simulink model "Two_Attitude_Estimation_ekf"  (R2021a)
settings: Solver=FixedStepAuto  StartTime=0.0  StopTime=200  FixedStep=Ts  RelTol=1e-5
values from neighbouring files (symbols this model uses):
  accel_filter_coef = [    0.0264    0.1405    0.3331    0.3331    0.1405    0.0264]    [quad_params_ekf.m]
  g = ref_acc(3)    [ekf_measurement_jacobian.m]    (also in quad_params_ekf.m = 9.81)
  gyro_filter_den = [ 1.0000    2.2287    2.5245    1.5773    0.5410    0.0796]    [quad_params_ekf.m]
  gyro_filter_num = [ 0.2821    1.2725    2.4208    2.4208    1.2725    0.2821]    [quad_params_ekf.m]
  I = [     0.005831943165131                   0                   0 ... (first row only)    [quad_params_ekf.m]
  Kd_rates = [0.05,0.05,0.1]'    [quad_params_ekf.m]
  Kd_vel = [0.8,0.8,0.3]'    [quad_params_ekf.m]
  Ki_vel = [0.1,0.1,0.1]'    [quad_params_ekf.m]
  km = 1.2e-7    (= 1.2e-07)    [quad_params_ekf.m]
  Kp_att = [6,6,6]'    [quad_params_ekf.m]
  Kp_pos = [7,7,3]'    [quad_params_ekf.m]
  Kp_rates = [10,10,10]'    [quad_params_ekf.m]
  Kp_vel = [3,3,5]'    [quad_params_ekf.m]
  kt = 0.9e-5    (= 9e-06)    [quad_params_ekf.m]
  L = 0.2    [quad_params_ekf.m]
  m = 0.9272    [quad_params_ekf.m]
  P_init = 0.01*eye(7)    [quad_params_ekf.m]
  Q = diag([0.015,0.0150,0.0150,0.0150,0.001,0.001,0.001])    [quad_params_ekf.m]
  q_init = [1;0;0;0]    [quad_params_ekf.m]
  R = diag([0.35,0.35,0.35,0.05,0.05,0.05])    [quad_params_ekf.m]
  rate_p_max = 3.5    [quad_params_ekf.m]
  thrust_max = thrust_max_per_motor*4    (= 32)    [quad_params_ekf.m]
  thrust_max_per_motor = 8    [quad_params_ekf.m]
  tilt_max = pi/6    (= 0.523598775598)    [quad_params_ekf.m]
  TQ_max_per_motor = km*(w_max.^2)    [quad_params_ekf.m]
  Ts = 0.001    [ekf_process_jacobian.m]    (also in ekf_process_model.m; quad_params_ekf.m)
  Ts_IMU = 0.001    [quad_params_ekf.m]
  Vb_init = [0;0;0]    [quad_params_ekf.m]
  vel_xy_max = 15    [quad_params_ekf.m]
  vel_z_max = 10    [quad_params_ekf.m]
  wb_init = [0;0;0]    [quad_params_ekf.m]
  x_0 = [1 0 0 0 0 0 0]'    [quad_params_ekf.m]
  Xe_init = [0;0;0]    [quad_params_ekf.m]
undefined symbols (not defined in the file or in its folder): IMU, p, pm_0, sigbuilder_block, Vm_0, xme_0
libraries: aerolibutil x8, simulink_extras x8, sharedtransform x7, sharedutil x6, simulink x4, pid_lib x3, aerolibcommonsys x3, aerolibnavsys x2, dspstat3 x2, mspsensorlib x1, aerolibnav x1, dspmtrx3 x1
(part 2 of 4)

== system Two_Attitude_Estimation_ekf/Thrust to attitude ==
  note: Thrust vector and Yaw to Attitude and total Thrust
  thrust_sp : Inport
  yaw_sp : Inport  Port=2
  Bus Creator : BusCreator  Inputs=3
  Demux4 : Demux  Outputs=3
  Direction Cosine Matrix to Quaternions : sharedtransform/Direction Cosine Matrix  to Quaternions  aMode=0  action=None  tolerance=eps(2)
      settings: SourceProductBaseCode=AE,PW,DR,MT,UV,VE
  MATLAB Function4 : MATLAB Function  TreatAsAtomicUnit=on
  Quaternions to Rotation Angles : sharedtransform/Quaternions to Rotation Angles  rotationOrder=ZYX  aMode=aMode
      settings: SourceProductBaseCode=AE,PW,DR,MT,UV,VE
  Scope1 : Scope
  Scope2 : Scope
  To Workspace : ToWorkspace  VariableName=thrust_unit_dir  SaveFormat=Timeseries  SampleTime=-1
  To Workspace1 : ToWorkspace  VariableName=thrust_mag  SaveFormat=Timeseries  SampleTime=-1
  thrust_mag : Outport
  q_cmd : Outport  Port=2
  euler_cmd : Outport  Port=3
  wires:
  thrust_sp/1 -> Scope1/1, MATLAB Function4/1(thrust_sp)  "thrust_cmd"
  MATLAB Function4/1(R_sp) -> To Workspace/1, Direction Cosine Matrix to Quaternions/1
  MATLAB Function4/2(thrust_mag) -> thrust_mag/1, To Workspace1/1
  Direction Cosine Matrix to Quaternions/1 -> q_cmd/1, Quaternions to Rotation Angles/1
  yaw_sp/1 -> MATLAB Function4/2(yaw_sp)  "yaw_cmd"
  Demux4/1 -> Bus Creator/1  "yaw"
  Demux4/3 -> Bus Creator/3  "roll"
  Bus Creator/1 -> Scope2/1, euler_cmd/1
  Demux4/2 -> Bus Creator/2  "pitch"
  Quaternions to Rotation Angles/1 -> Demux4/1

== system Two_Attitude_Estimation_ekf/Trajectory command ==
  Altitude : Subsystem  VariantControl=1
  Ground : Subsystem  VariantControl=0
  Position Trajectory : Subsystem  VariantControl=5
  Test to visualize thrust dir : Subsystem  VariantControl=6
  X Sine : Subsystem  VariantControl=4
  X ramp : Subsystem  VariantControl=9
  X square : Subsystem  VariantControl=7
  Y Sine : Subsystem  VariantControl=3
  Y ramp : Subsystem  VariantControl=8
  Yaw Sine : Subsystem  VariantControl=2
  Yaw steps : Subsystem  VariantControl=10
  Z : Outport
  Y : Outport  Port=2
  X : Outport  Port=3
  Yaw : Outport  Port=4
  CMD_VEC : Outport  Port=5

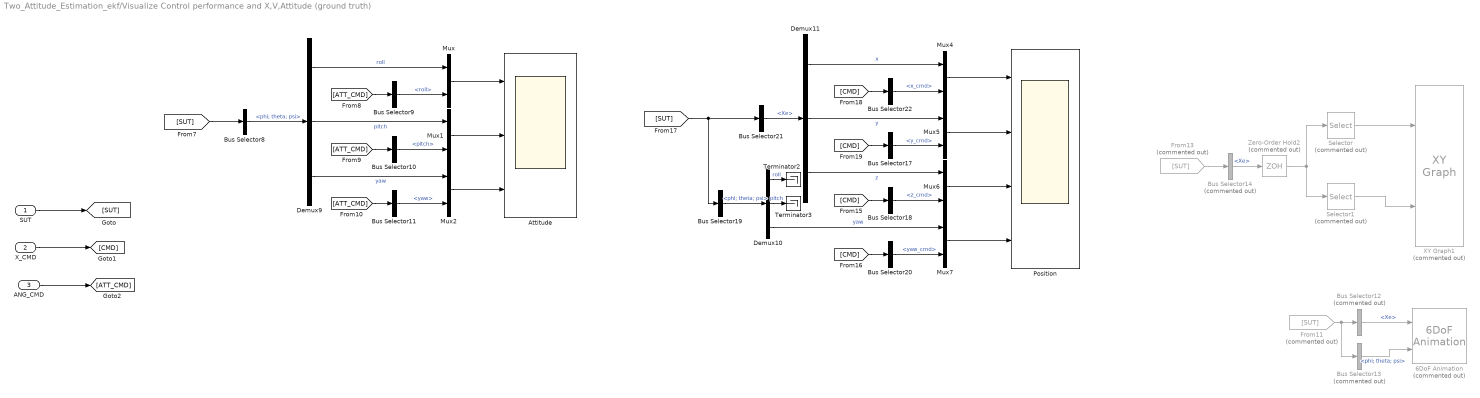
== system Two_Attitude_Estimation_ekf/Visualize Control performance and X,V,Attitude (ground truth) ==
  SUT : Inport
  X_CMD : Inport  Port=2
  ANG_CMD : Inport  Port=3
  6DoF Animation : aerolibanim/6DoF Animation  Commented=on  u1=[-20 20 -20 20 -20 20]  u2=0.05  u3=0.5  u4=[-5 -5 0 5]  u5=Fly alongside  u6=[0 0 0]  u7=10  u8=on
  "Attitude " : Scope  NumInputPorts=3
  Bus Selector10 : BusSelector  OutputSignals=pitch
  Bus Selector11 : BusSelector  OutputSignals=yaw
  Bus Selector12 : BusSelector  Commented=on  OutputSignals=Xe
  Bus Selector13 : BusSelector  Commented=on  OutputSignals=phi; theta; psi
  Bus Selector14 : BusSelector  Commented=on  OutputSignals=Xe
  Bus Selector17 : BusSelector  OutputSignals=y_cmd
  Bus Selector18 : BusSelector  OutputSignals=z_cmd
  Bus Selector19 : BusSelector  OutputSignals=phi; theta; psi
  Bus Selector20 : BusSelector  OutputSignals=yaw_cmd
  Bus Selector21 : BusSelector  OutputSignals=Xe
  Bus Selector22 : BusSelector  OutputSignals=x_cmd
  Bus Selector8 : BusSelector  OutputSignals=phi; theta; psi
  Bus Selector9 : BusSelector  OutputSignals=roll
  Demux10 : Demux  Outputs=3
  Demux11 : Demux  Outputs=3
  Demux9 : Demux  Outputs=3
  From11 : From  Commented=on  GotoTag=SUT
  From13 : From  Commented=on  GotoTag=SUT
  Mux{,1..2,4..7} (7 alike) : Mux  Inputs=2
  Position : Scope  NumInputPorts=4
  Selector : Selector  Commented=on  InputPortWidth=3  IndexOptions=Index vector (dialog)  Indices=1  OutputSizes=1
  Selector1 : Selector  Commented=on  InputPortWidth=3  IndexOptions=Index vector (dialog)  Indices=2  OutputSizes=1
  Terminator2 : Terminator
  Terminator3 : Terminator
  XY Graph1 : simulink/Sinks/XY Graph  Commented=on  xmin=-1  xmax=30  ymin=-1  ymax=35  st=-1
  Zero-Order Hold2 : ZeroOrderHold  Commented=on  SampleTime=0.1
  wires:
  SUT/1 -> [SUT]
  X_CMD/1 -> [CMD]
  [SUT] -> Bus Selector8/1
  Demux9/2 -> Mux1/1  "pitch"
  Demux9/1 -> Mux/1  "roll"
  Bus Selector8/1 -> Demux9/1  "<phi; theta; psi>"
  Mux/1 -> "Attitude "/1
  Mux1/1 -> "Attitude "/2
  Mux2/1 -> "Attitude "/3
  Demux9/3 -> Mux2/1  "yaw"
  [ATT_CMD] -> Bus Selector9/1
  Bus Selector9/1 -> Mux/2  "<roll>"
  [ATT_CMD] -> Bus Selector10/1
  Bus Selector10/1 -> Mux1/2  "<pitch>"
  [ATT_CMD] -> Bus Selector11/1
  Bus Selector11/1 -> Mux2/2  "<yaw>"
  From13/1 -> Bus Selector14/1
  Bus Selector14/1 -> Zero-Order Hold2/1  "<Xe>"
  Zero-Order Hold2/1 -> Selector1/1, Selector/1
  Demux10/3 -> Mux7/1  "yaw"
  Mux7/1 -> Position/4
  Demux11/1 -> Mux4/1  "x"
  [CMD] -> Bus Selector20/1
  Bus Selector20/1 -> Mux7/2  "<yaw_cmd>"
  [CMD] -> Bus Selector17/1
  [SUT] -> Bus Selector21/1, Bus Selector19/1
  Demux10/2 -> Terminator3/1  "pitch"
  Mux6/1 -> Position/3
  Bus Selector19/1 -> Demux10/1  "<phi; theta; psi>"
  Demux10/1 -> Terminator2/1  "roll"
  Demux11/2 -> Mux5/1  "y"
  Bus Selector17/1 -> Mux5/2  "<y_cmd>"
  Mux4/1 -> Position/1
  Demux11/3 -> Mux6/1  "z"
  [CMD] -> Bus Selector22/1
  Mux5/1 -> Position/2
  Bus Selector22/1 -> Mux4/2  "<x_cmd>"
  Bus Selector18/1 -> Mux6/2  "<z_cmd>"
  [CMD] -> Bus Selector18/1
  Bus Selector21/1 -> Demux11/1  "<Xe>"
  ANG_CMD/1 -> [ATT_CMD]
  Selector/1 -> XY Graph1/1
  Selector1/1 -> XY Graph1/2
  From11/1 -> Bus Selector13/1, Bus Selector12/1
  Bus Selector12/1 -> 6DoF Animation/1  "<Xe>"
  Bus Selector13/1 -> 6DoF Animation/2  "<phi; theta; psi>"

== system Two_Attitude_Estimation_ekf/Control allocation and motor control/Ideal Actuators with allocation ==
  THRUST_CMD : Inport
  TQ_Roll_CMD : Inport  Port=2
  TQ_Pitch_CMD : Inport  Port=3
  TQ_Yaw_CMD : Inport  Port=4
  Control allocation : Subsystem
  Perfect actuators : Subsystem  VariantControl=Choice2
  Thrust : Outport
  Mx : Outport  Port=2
  My : Outport  Port=3
  Mz : Outport  Port=4
  T_actual : Outport  Port=5
  w_mot_actual : Outport  Port=6
  wires:
  Control allocation/1(w_command) -> Perfect actuators/1(w_cmd)
  THRUST_CMD/1 -> Control allocation/1(THRUST_CMD)
  TQ_Pitch_CMD/1 -> Control allocation/3(TQ_Pitch_CMD)
  TQ_Roll_CMD/1 -> Control allocation/2(TQ_Roll_CMD)
  TQ_Yaw_CMD/1 -> Control allocation/4(TQ_Yaw_CMD)
  Perfect actuators/5(T_actual) -> T_actual/1
  Perfect actuators/6(w_mot_actual) -> w_mot_actual/1
  Perfect actuators/3(My) -> My/1
  Perfect actuators/2(Mx) -> Mx/1
  Perfect actuators/4(Mz) -> Mz/1
  Perfect actuators/1(Thrust) -> Thrust/1

== system Two_Attitude_Estimation_ekf/Control allocation and motor control/Ideal Actuattion (direct transfer) ==
  THRUST_CMD : Inport
  TQ_Roll_CMD : Inport  Port=2
  TQ_Pitch_CMD : Inport  Port=3
  TQ_Yaw_CMD : Inport  Port=4
  Mux : Mux
  Zero : Constant  Value=[0;0;0;0]  OutDataTypeStr=Inherit: Inherit via back propagation
  Thrust : Outport
  Mx : Outport  Port=2
  My : Outport  Port=3
  Mz : Outport  Port=4
  T_actual : Outport  Port=5
  w_mot_actual : Outport  Port=6
  wires:
  Zero/1 -> w_mot_actual/1
  TQ_Pitch_CMD/1 -> Mux/3, My/1
  TQ_Roll_CMD/1 -> Mux/2, Mx/1
  TQ_Yaw_CMD/1 -> Mux/4, Mz/1
  THRUST_CMD/1 -> Mux/1, Thrust/1
  Mux/1 -> T_actual/1

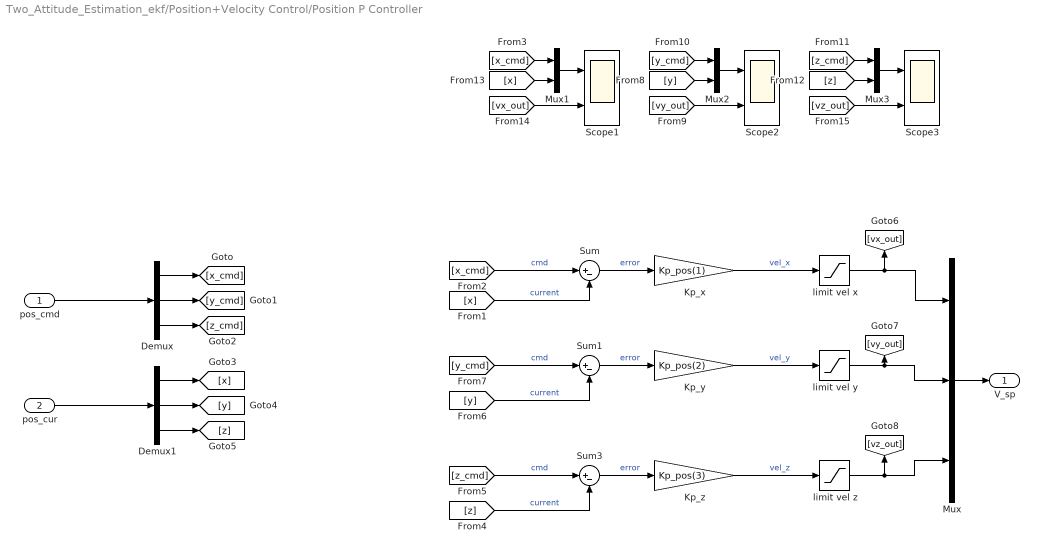
== system Two_Attitude_Estimation_ekf/Position+Velocity Control/Position P Controller ==
  pos_cmd : Inport
  pos_cur : Inport  Port=2
  Demux : Demux  Outputs=3
  Demux1 : Demux  Outputs=3
  Kp_x : Gain  Gain=Kp_pos(1)
  Kp_y : Gain  Gain=Kp_pos(2)
  Kp_z : Gain  Gain=Kp_pos(3)
  Mux : Mux  Inputs=3
  Mux1 : Mux  Inputs=2
  Mux2 : Mux  Inputs=2
  Mux3 : Mux  Inputs=2
  Scope1 : Scope  NumInputPorts=2
  Scope2 : Scope  NumInputPorts=2
  Scope3 : Scope  NumInputPorts=2
  Sum : Sum  Inputs=|+-
  Sum1 : Sum  Inputs=|+-
  Sum3 : Sum  Inputs=|+-
  limit vel x : Saturate  UpperLimit=vel_xy_max  LowerLimit=-vel_xy_max
  limit vel y : Saturate  UpperLimit=vel_xy_max  LowerLimit=-vel_xy_max
  limit vel z : Saturate  UpperLimit=vel_z_max  LowerLimit=-vel_z_max
  V_sp : Outport
  wires:
  pos_cmd/1 -> Demux/1
  pos_cur/1 -> Demux1/1
  Demux/1 -> [x_cmd]
  Demux/2 -> [y_cmd]
  Demux/3 -> [z_cmd]
  Demux1/1 -> [x]
  Demux1/3 -> [z]
  Demux1/2 -> [y]
  [x_cmd] -> Sum/1  "cmd"
  Sum/1 -> Kp_x/1  "error"
  Mux/1 -> V_sp/1
  Kp_x/1 -> limit vel x/1  "vel_x"
  [x] -> Sum/2  "current"
  [z_cmd] -> Sum3/1  "cmd"
  [z] -> Sum3/2  "current"
  Sum3/1 -> Kp_z/1  "error"
  [y_cmd] -> Sum1/1  "cmd"
  [y] -> Sum1/2  "current"
  Sum1/1 -> Kp_y/1  "error"
  Kp_z/1 -> limit vel z/1  "vel_z"
  limit vel x/1 -> [vx_out], Mux/1
  Kp_y/1 -> limit vel y/1  "vel_y"
  limit vel y/1 -> [vy_out], Mux/2
  limit vel z/1 -> [vz_out], Mux/3
  [x_cmd] -> Mux1/1
  Mux1/1 -> Scope1/1
  [vx_out] -> Scope1/2
  [x] -> Mux1/2
  [y_cmd] -> Mux2/1
  Mux2/1 -> Scope2/1
  [vy_out] -> Scope2/2
  [y] -> Mux2/2
  [z_cmd] -> Mux3/1
  Mux3/1 -> Scope3/1
  [vz_out] -> Scope3/2
  [z] -> Mux3/2

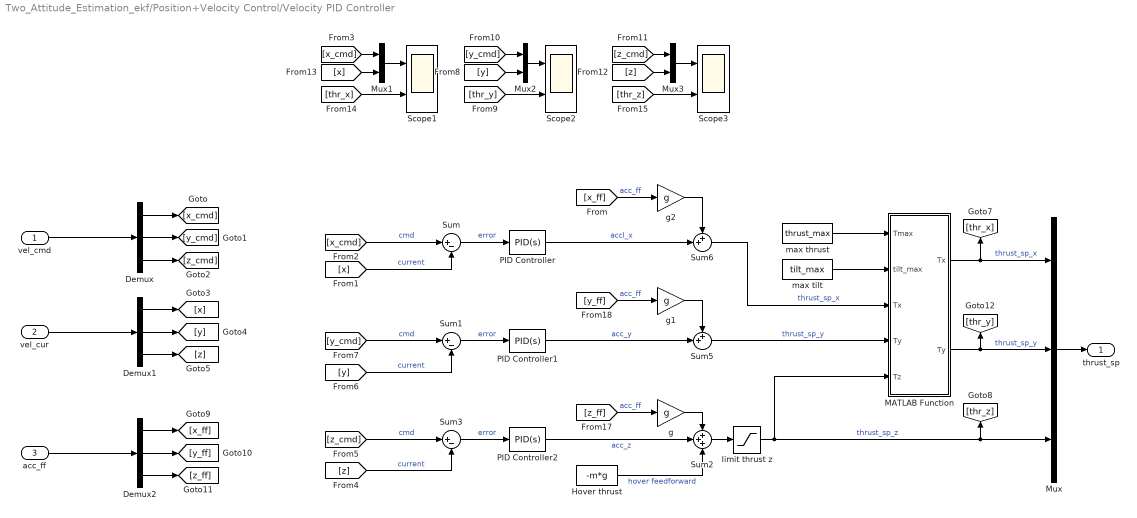
== system Two_Attitude_Estimation_ekf/Position+Velocity Control/Velocity PID Controller ==
  vel_cmd : Inport
  vel_cur : Inport  Port=2
  acc_ff : Inport  Port=3
  Demux : Demux  Outputs=3
  Demux1 : Demux  Outputs=3
  Demux2 : Demux  Outputs=3
  Hover thrust : Constant  Value=-m*g
  MATLAB Function : MATLAB Function  TreatAsAtomicUnit=on
  Mux : Mux  Inputs=3
  Mux1 : Mux  Inputs=2
  Mux2 : Mux  Inputs=2
  Mux3 : Mux  Inputs=2
  PID Controller : pid_lib/PID Controller  Controller=PID  Form=Parallel  TimeDomain=Continuous-time  UseExternalTs=off  SampleTime=-1  IntegratorMethod=Forward Euler  FilterMethod=Forward Euler  ControllerParametersSource=internal  P=Kp_vel(1)  I=Ki_vel(1)  D=Kd_vel(1)  UseFilter=on  N=100  TunerSelectOption=Transfer Function Based (PID Tuner App)  InitialConditionSource=internal  InitialConditionForIntegrator=0  InitialConditionForFilter=0  DifferentiatorICPrevScaledInput=0  ExternalReset=none  TrackingMode=off  Kt=1  LimitOutput=off  SatLimitsSource=internal  UpperSaturationLimit=inf  LowerSaturationLimit=-inf  LinearizeAsGain=on  AntiWindupMode=none  Kb=1  POutMin=[]  POutMax=[]  IOutMin=[]  IOutMax=[]  DOutMin=[]  DOutMax=[]  NOutMin=[]  NOutMax=[]  SumOutMin=[]  SumOutMax=[]  SaturationOutMin=[]  SaturationOutMax=[]  PParamMin=[]  PParamMax=[]  IParamMin=[]  IParamMax=[]  DParamMin=[]  DParamMax=[]  NParamMin=[]  NParamMax=[]  KbParamMin=[]  KbParamMax=[]  KtParamMin=[]  KtParamMax=[]  KbOutMin=[]  KbOutMax=[]  KtOutMin=[]  KtOutMax=[]  IntegratorOutMin=[]  IntegratorOutMax=[]  FilterOutMin=[]  FilterOutMax=[]  SumI1OutMin=[]  SumI1OutMax=[]  SumI2OutMin=[]  SumI2OutMax=[]  SumI3OutMin=[]  SumI3OutMax=[]  SumI4OutMin=[]  SumI4OutMax=[]  SumDOutMin=[]  SumDOutMax=[]  DifferentiatorOutMin=[]  DifferentiatorOutMax=[]  FilterDiffOutCoefMin=[]  FilterDiffOutCoefMax=[]  ReciprocalOutMin=[]  ReciprocalOutMax=[]  SumDenOutMin=[]  SumDenOutMax=[]  SumNumOutMin=[]  SumNumOutMax=[]  DivideOutMin=[]  DivideOutMax=[]  UdiffTsProdOutMin=[]  UdiffTsProdOutMax=[]  NTsProdOutMin=[]  NTsProdOutMax=[]  UintegralTsProdOutMin=[]  UintegralTsProdOutMax=[]  UngainTsProdOutMin=[]  UngainTsProdOutMax=[]  IntegratorContinuousStateAttributes=''  IntegratorStateMustResolveToSignalObject=off  IntegratorRTWStateStorageClass=Auto  FilterContinuousStateAttributes=''  FilterStateMustResolveToSignalObject=off  FilterRTWStateStorageClass=Auto  ParallelPVariant=InternalParameters  IdealPVariant=Disabled  IVariant=InternalParameters  DVariant=InternalParameters  IntegratorVariant=Continuous  SatVariant=Disabled  AWVariant=Passthrough  PCopyVariant=Disabled  TRVariant=Disabled  FdbkBlocksVariant=Forward  IdealPFdbkVariant=Disabled  SatFdbkVariant=Disabled  DerivativeFilterVariant=ContFilter  NVariant=InternalParameters  NCopyVariant=Disabled  FilterICVariant=InternalICsFilter  IntegratorICVariant=InternalICs  ExternalResetVariant=Disabled  TRSumVariant=Passthrough  SumFdbkVariant=Disabled  SumVariant=Sum_PID  TsampFilterVariant=InternalTs  TsampNgainVariant=Passthrough  TsampIntegralVariant=Passthrough  ExternalSaturationOutDataTypeStr=Inherit: Same as second input
  PID Controller1 : pid_lib/PID Controller  Controller=PID  Form=Parallel  TimeDomain=Continuous-time  UseExternalTs=off  SampleTime=-1  IntegratorMethod=Forward Euler  FilterMethod=Forward Euler  ControllerParametersSource=internal  P=Kp_vel(2)  I=Ki_vel(2)  D=Kd_vel(2)  UseFilter=on  N=100  TunerSelectOption=Transfer Function Based (PID Tuner App)  InitialConditionSource=internal  InitialConditionForIntegrator=0  InitialConditionForFilter=0  DifferentiatorICPrevScaledInput=0  ExternalReset=none  TrackingMode=off  Kt=1  LimitOutput=off  SatLimitsSource=internal  UpperSaturationLimit=inf  LowerSaturationLimit=-inf  LinearizeAsGain=on  AntiWindupMode=none  Kb=1  POutMin=[]  POutMax=[]  IOutMin=[]  IOutMax=[]  DOutMin=[]  DOutMax=[]  NOutMin=[]  NOutMax=[]  SumOutMin=[]  SumOutMax=[]  SaturationOutMin=[]  SaturationOutMax=[]  PParamMin=[]  PParamMax=[]  IParamMin=[]  IParamMax=[]  DParamMin=[]  DParamMax=[]  NParamMin=[]  NParamMax=[]  KbParamMin=[]  KbParamMax=[]  KtParamMin=[]  KtParamMax=[]  KbOutMin=[]  KbOutMax=[]  KtOutMin=[]  KtOutMax=[]  IntegratorOutMin=[]  IntegratorOutMax=[]  FilterOutMin=[]  FilterOutMax=[]  SumI1OutMin=[]  SumI1OutMax=[]  SumI2OutMin=[]  SumI2OutMax=[]  SumI3OutMin=[]  SumI3OutMax=[]  SumI4OutMin=[]  SumI4OutMax=[]  SumDOutMin=[]  SumDOutMax=[]  DifferentiatorOutMin=[]  DifferentiatorOutMax=[]  FilterDiffOutCoefMin=[]  FilterDiffOutCoefMax=[]  ReciprocalOutMin=[]  ReciprocalOutMax=[]  SumDenOutMin=[]  SumDenOutMax=[]  SumNumOutMin=[]  SumNumOutMax=[]  DivideOutMin=[]  DivideOutMax=[]  UdiffTsProdOutMin=[]  UdiffTsProdOutMax=[]  NTsProdOutMin=[]  NTsProdOutMax=[]  UintegralTsProdOutMin=[]  UintegralTsProdOutMax=[]  UngainTsProdOutMin=[]  UngainTsProdOutMax=[]  IntegratorContinuousStateAttributes=''  IntegratorStateMustResolveToSignalObject=off  IntegratorRTWStateStorageClass=Auto  FilterContinuousStateAttributes=''  FilterStateMustResolveToSignalObject=off  FilterRTWStateStorageClass=Auto  ParallelPVariant=InternalParameters  IdealPVariant=Disabled  IVariant=InternalParameters  DVariant=InternalParameters  IntegratorVariant=Continuous  SatVariant=Disabled  AWVariant=Passthrough  PCopyVariant=Disabled  TRVariant=Disabled  FdbkBlocksVariant=Forward  IdealPFdbkVariant=Disabled  SatFdbkVariant=Disabled  DerivativeFilterVariant=ContFilter  NVariant=InternalParameters  NCopyVariant=Disabled  FilterICVariant=InternalICsFilter  IntegratorICVariant=InternalICs  ExternalResetVariant=Disabled  TRSumVariant=Passthrough  SumFdbkVariant=Disabled  SumVariant=Sum_PID  TsampFilterVariant=InternalTs  TsampNgainVariant=Passthrough  TsampIntegralVariant=Passthrough  ExternalSaturationOutDataTypeStr=Inherit: Same as second input
  PID Controller2 : pid_lib/PID Controller  Controller=PID  Form=Parallel  TimeDomain=Continuous-time  UseExternalTs=off  SampleTime=-1  IntegratorMethod=Forward Euler  FilterMethod=Forward Euler  ControllerParametersSource=internal  P=Kp_vel(3)  I=Ki_vel(3)  D=Kd_vel(3)  UseFilter=on  N=100  TunerSelectOption=Transfer Function Based (PID Tuner App)  InitialConditionSource=internal  InitialConditionForIntegrator=0  InitialConditionForFilter=0  DifferentiatorICPrevScaledInput=0  ExternalReset=none  TrackingMode=off  Kt=1  LimitOutput=off  SatLimitsSource=internal  UpperSaturationLimit=inf  LowerSaturationLimit=-inf  LinearizeAsGain=on  AntiWindupMode=none  Kb=1  POutMin=[]  POutMax=[]  IOutMin=[]  IOutMax=[]  DOutMin=[]  DOutMax=[]  NOutMin=[]  NOutMax=[]  SumOutMin=[]  SumOutMax=[]  SaturationOutMin=[]  SaturationOutMax=[]  PParamMin=[]  PParamMax=[]  IParamMin=[]  IParamMax=[]  DParamMin=[]  DParamMax=[]  NParamMin=[]  NParamMax=[]  KbParamMin=[]  KbParamMax=[]  KtParamMin=[]  KtParamMax=[]  KbOutMin=[]  KbOutMax=[]  KtOutMin=[]  KtOutMax=[]  IntegratorOutMin=[]  IntegratorOutMax=[]  FilterOutMin=[]  FilterOutMax=[]  SumI1OutMin=[]  SumI1OutMax=[]  SumI2OutMin=[]  SumI2OutMax=[]  SumI3OutMin=[]  SumI3OutMax=[]  SumI4OutMin=[]  SumI4OutMax=[]  SumDOutMin=[]  SumDOutMax=[]  DifferentiatorOutMin=[]  DifferentiatorOutMax=[]  FilterDiffOutCoefMin=[]  FilterDiffOutCoefMax=[]  ReciprocalOutMin=[]  ReciprocalOutMax=[]  SumDenOutMin=[]  SumDenOutMax=[]  SumNumOutMin=[]  SumNumOutMax=[]  DivideOutMin=[]  DivideOutMax=[]  UdiffTsProdOutMin=[]  UdiffTsProdOutMax=[]  NTsProdOutMin=[]  NTsProdOutMax=[]  UintegralTsProdOutMin=[]  UintegralTsProdOutMax=[]  UngainTsProdOutMin=[]  UngainTsProdOutMax=[]  IntegratorContinuousStateAttributes=''  IntegratorStateMustResolveToSignalObject=off  IntegratorRTWStateStorageClass=Auto  FilterContinuousStateAttributes=''  FilterStateMustResolveToSignalObject=off  FilterRTWStateStorageClass=Auto  ParallelPVariant=InternalParameters  IdealPVariant=Disabled  IVariant=InternalParameters  DVariant=InternalParameters  IntegratorVariant=Continuous  SatVariant=Disabled  AWVariant=Passthrough  PCopyVariant=Disabled  TRVariant=Disabled  FdbkBlocksVariant=Forward  IdealPFdbkVariant=Disabled  SatFdbkVariant=Disabled  DerivativeFilterVariant=ContFilter  NVariant=InternalParameters  NCopyVariant=Disabled  FilterICVariant=InternalICsFilter  IntegratorICVariant=InternalICs  ExternalResetVariant=Disabled  TRSumVariant=Passthrough  SumFdbkVariant=Disabled  SumVariant=Sum_PID  TsampFilterVariant=InternalTs  TsampNgainVariant=Passthrough  TsampIntegralVariant=Passthrough  ExternalSaturationOutDataTypeStr=Inherit: Same as second input
  Scope1 : Scope  NumInputPorts=2
  Scope2 : Scope  NumInputPorts=2
  Scope3 : Scope  NumInputPorts=2
  Sum : Sum  Inputs=|+-
  Sum1 : Sum  Inputs=|+-
  Sum2 : Sum  Inputs=+++
  Sum3 : Sum  Inputs=|+-
  Sum5 : Sum  Inputs=++|
  Sum6 : Sum  Inputs=++|
  g : Gain  Gain=g
  g1 : Gain  Gain=g
  g2 : Gain  Gain=g
  limit thrust z : Saturate  UpperLimit=thrust_max  LowerLimit=-thrust_max
  max thrust : Constant  Value=thrust_max
  max tilt : Constant  Value=tilt_max
  thrust_sp : Outport
  wires:
  vel_cmd/1 -> Demux/1
  vel_cur/1 -> Demux1/1
  Demux/1 -> [x_cmd]
  Demux/2 -> [y_cmd]
  Demux/3 -> [z_cmd]
  Demux1/1 -> [x]
  Demux1/3 -> [z]
  Demux1/2 -> [y]
  [x_cmd] -> Sum/1  "cmd"
  [thr_x] -> Scope1/2
  Sum/1 -> PID Controller/1  "error"
  Mux/1 -> thrust_sp/1
  [x] -> Sum/2  "current"
  [z_cmd] -> Sum3/1  "cmd"
  [z] -> Sum3/2  "current"
  Sum3/1 -> PID Controller2/1  "error"
  [y_cmd] -> Sum1/1  "cmd"
  [y] -> Sum1/2  "current"
  Sum1/1 -> PID Controller1/1  "error"
  limit thrust z/1 -> [thr_z], Mux/3, MATLAB Function/5(Tz)  "thrust_sp_z"
  Demux2/3 -> [z_ff]
  acc_ff/1 -> Demux2/1
  Demux2/2 -> [y_ff]
  Demux2/1 -> [x_ff]
  Hover thrust/1 -> Sum2/3  "hover feedforward"
  PID Controller2/1 -> Sum2/2  "acc_z"
  [z_ff] -> g/1  "acc_ff"
  g/1 -> Sum2/1
  [y_ff] -> g1/1  "acc_ff"
  PID Controller1/1 -> Sum5/2  "acc_y"
  g1/1 -> Sum5/1
  g2/1 -> Sum6/1
  [x_ff] -> g2/1  "acc_ff"
  PID Controller/1 -> Sum6/2  "accl_x"
  Sum2/1 -> limit thrust z/1
  max thrust/1 -> MATLAB Function/1(Tmax)
  max tilt/1 -> MATLAB Function/2(tilt_max)
  Mux1/1 -> Scope1/1
  [x_cmd] -> Mux1/1
  [x] -> Mux1/2
  [y_cmd] -> Mux2/1
  Mux2/1 -> Scope2/1
  [thr_y] -> Scope2/2
  [y] -> Mux2/2
  [z_cmd] -> Mux3/1
  Mux3/1 -> Scope3/1
  [thr_z] -> Scope3/2
  [z] -> Mux3/2
  MATLAB Function/1(Tx) -> Mux/1, [thr_x]  "thrust_sp_x"
  Sum6/1 -> MATLAB Function/3("Tx ")  "thrust_sp_x"
  Sum5/1 -> MATLAB Function/4("Ty ")  "thrust_sp_y"
  MATLAB Function/2(Ty) -> [thr_y], Mux/2  "thrust_sp_y"

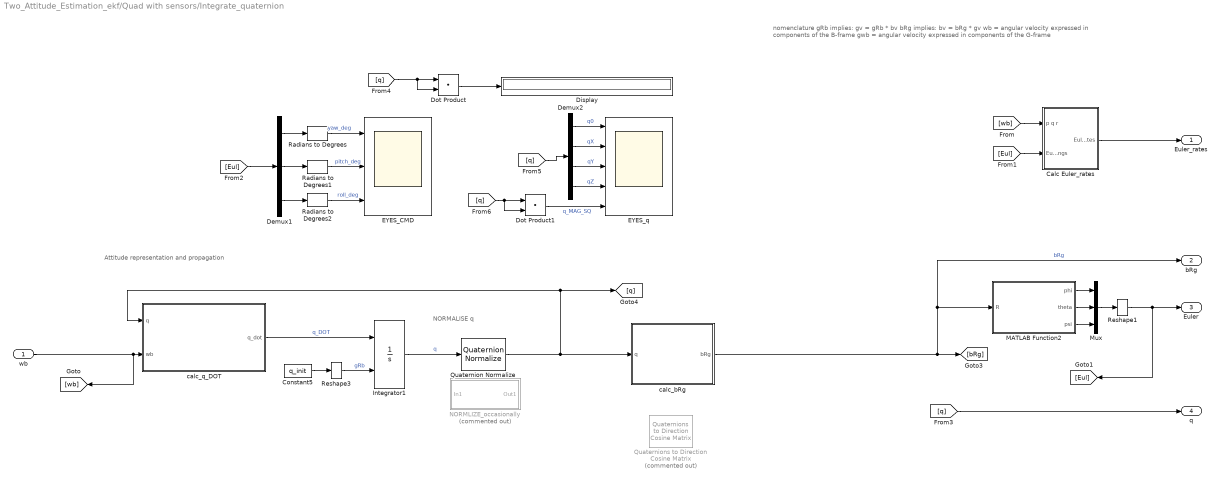
== system Two_Attitude_Estimation_ekf/Quad with sensors/Integrate_quaternion ==
  note: Attitude representation and propagation
  note: nomenclature
      | gRb implies: gv = gRb * bv
      | bRg implies: bv = bRg * gv
      |
      | wb = angular velocity expressed in components of the B-frame
      | gwb = angular velocity expressed in components of the G-frame
  note: NORMALISE q
  wb : Inport
  Calc Euler_rates : Subsystem
  Constant5 : Constant  Value=q_init  OutDataTypeStr=Inherit: Inherit via back propagation
  Demux1 : Demux  Outputs=3
  Demux2 : Demux
  Display : Display
  Dot Product : DotProduct  InputSameDT=on  OutDataTypeStr=Inherit: Inherit via internal rule
  Dot Product1 : DotProduct  InputSameDT=on  OutDataTypeStr=Inherit: Inherit via internal rule
  EYES_CMD : Scope  NumInputPorts=3
  EYES_q : Scope  NumInputPorts=5
  Integrator1 : Integrator  InitialConditionSource=external
  MATLAB Function2 : MATLAB Function  TreatAsAtomicUnit=on
  Mux : Mux  Inputs=3
  NORMLIZE_occasionally : Subsystem  Commented=on
  Quaternion Normalize : sharedutil/Quaternion Normalize  aMode=aMode
      settings: SourceProductBaseCode=AE,PW,DR,MT,UV,VE
  Quaternions to Direction Cosine Matrix : sharedtransform/Quaternions to  Direction Cosine Matrix  Commented=on  aMode=aMode
      settings: SourceProductBaseCode=AE,PW,DR,MT,UV,VE
  Radians to Degrees : simulink_extras/Transformations/Radians to Degrees
  Radians to Degrees1 : simulink_extras/Transformations/Radians to Degrees
  Radians to Degrees2 : simulink_extras/Transformations/Radians to Degrees
  Reshape1 : Reshape  OutputDimensionality=Column vector (2-D)
  Reshape3 : Reshape  OutputDimensionality=Column vector (2-D)
  calc_bRg : MATLAB Function  TreatAsAtomicUnit=on
  calc_q_DOT : MATLAB Function  TreatAsAtomicUnit=on
  Euler_rates : Outport
  bRg : Outport  Port=2
  Euler : Outport  Port=3
  q : Outport  Port=4
  wires:
  Calc Euler_rates/1(Euler_rates) -> Euler_rates/1
  [Eul] -> Demux1/1
  Demux1/2 -> Radians to Degrees1/1
  Demux1/3 -> Radians to Degrees2/1
  Radians to Degrees2/1 -> EYES_CMD/3  "roll_deg"
  Radians to Degrees1/1 -> EYES_CMD/2  "pitch_deg"
  Radians to Degrees/1 -> EYES_CMD/1  "yaw_deg"
  Demux1/1 -> Radians to Degrees/1
  [Eul] -> Calc Euler_rates/2(Euler_angs)
  [wb] -> Calc Euler_rates/1("p q r ")
  Reshape1/1 -> [Eul], Euler/1
  Mux/1 -> Reshape1/1
  MATLAB Function2/3(psi) -> Mux/3
  MATLAB Function2/2(theta) -> Mux/2
  MATLAB Function2/1(phi) -> Mux/1
  Demux2/3 -> EYES_q/3  "qY"
  [q] -> Demux2/1
  Demux2/2 -> EYES_q/2  "qX"
  Demux2/1 -> EYES_q/1  "q0"
  [q] -> Dot Product1/2, Dot Product1/1
  Demux2/4 -> EYES_q/4  "qZ"
  Dot Product1/1 -> EYES_q/5  "q_MAG_SQ"
  Dot Product/1 -> Display/1
  [q] -> Dot Product/2, Dot Product/1
  Integrator1/1 -> Quaternion Normalize/1  "q"
  Quaternion Normalize/1 -> calc_bRg/1(q), [q], calc_q_DOT/1(q)
  calc_bRg/1(bRg) -> bRg/1, MATLAB Function2/1(R), [bRg]  "bRg"
  calc_q_DOT/1(q_dot) -> Integrator1/1  "q_DOT"
  Constant5/1 -> Reshape3/1
  wb/1 -> calc_q_DOT/2(wb), [wb]
  Reshape3/1 -> Integrator1/2  "gRb"
  [q] -> q/1

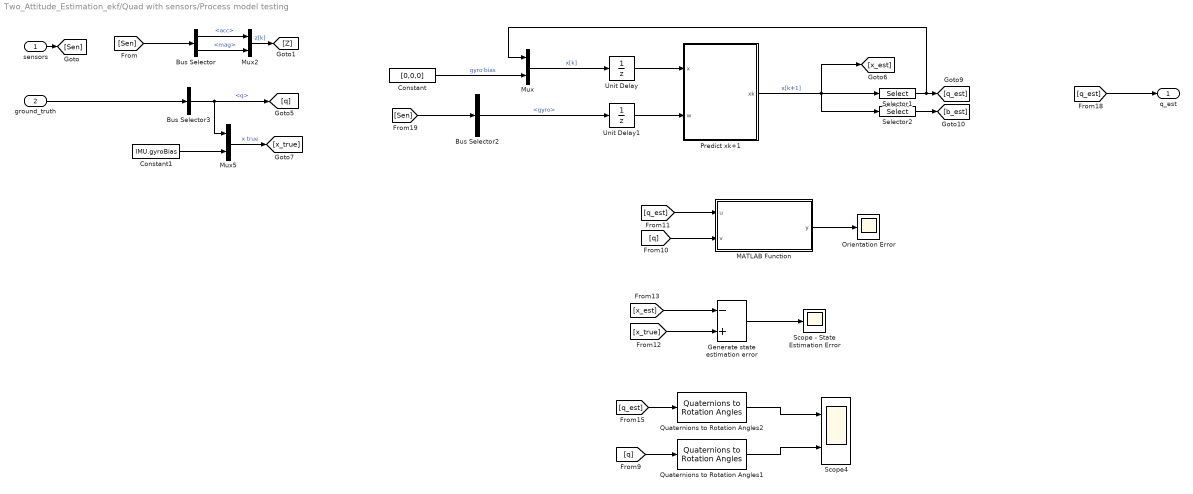
== system Two_Attitude_Estimation_ekf/Quad with sensors/Process model testing ==
  sensors : Inport
  ground_truth : Inport  Port=2
  Bus Selector : BusSelector  OutputSignals=acc,mag
  Bus Selector2 : BusSelector  OutputSignals=gyro
  Bus Selector3 : BusSelector  OutputSignals=q
  Constant : Constant  Value=[0,0,0]
  Constant1 : Constant  Value=IMU.gyroBias
  Generate state estimation error : Sum  Inputs=-+
  MATLAB Function : MATLAB Function  TreatAsAtomicUnit=on
  Mux : Mux  Inputs=2
  Mux2 : Mux  Inputs=2
  Mux5 : Mux  Inputs=2
  Orientation Error : Scope
  Predict xk+1 : MATLAB Function  TreatAsAtomicUnit=on
  Quaternions to Rotation Angles1 : sharedtransform/Quaternions to Rotation Angles  rotationOrder=ZYX  aMode=aMode
      settings: SourceProductBaseCode=AE,PW,DR,MT,UV,VE
  Quaternions to Rotation Angles2 : sharedtransform/Quaternions to Rotation Angles  rotationOrder=ZYX  aMode=aMode
      settings: SourceProductBaseCode=AE,PW,DR,MT,UV,VE
  Scope - State Estimation Error : Scope
  Scope4 : Scope  NumInputPorts=2
  Selector1 : Selector  InputPortWidth=7  IndexOptions=Index vector (dialog)  Indices=[1:4]  OutputSizes=1
  Selector2 : Selector  InputPortWidth=7  IndexOptions=Index vector (dialog)  Indices=[5:7]  OutputSizes=1
  Unit Delay : UnitDelay  InitialCondition=x_0  SampleTime=-1  HasFrameUpgradeWarning=on
  Unit Delay1 : UnitDelay  SampleTime=-1  HasFrameUpgradeWarning=on
  q_est : Outport
  wires:
  Bus Selector3/1 -> [q], Mux5/1  "<q>"
  [Sen] -> Bus Selector/1
  Bus Selector/1 -> Mux2/1  "<acc>"
  Bus Selector/2 -> Mux2/2  "<mag>"
  Quaternions to Rotation Angles2/1 -> Scope4/1
  Generate state estimation error/1 -> Scope - State Estimation Error/1
  MATLAB Function/1(y) -> Orientation Error/1
  Quaternions to Rotation Angles1/1 -> Scope4/2
  ground_truth/1 -> Bus Selector3/1
  sensors/1 -> [Sen]
  Mux2/1 -> [Z]  "z[k]"
  [q] -> Quaternions to Rotation Angles1/1
  [q] -> MATLAB Function/2(v)
  [q_est] -> MATLAB Function/1(u)
  [x_est] -> Generate state estimation error/1
  Mux5/1 -> [x_true]  "x true"
  Constant1/1 -> Mux5/2
  [x_true] -> Generate state estimation error/2
  [q_est] -> Quaternions to Rotation Angles2/1
  [q_est] -> q_est/1
  Mux/1 -> Unit Delay/1  "x[k]"
  Unit Delay/1 -> Predict xk+1/1(x)
  Selector1/1 -> [q_est], Mux/1
  Constant/1 -> Mux/2  "gyro bias"
  Unit Delay1/1 -> Predict xk+1/2(w)
  Predict xk+1/1(xk) -> [x_est], Selector2/1, Selector1/1  "x[k+1]"
  Bus Selector2/1 -> Unit Delay1/1  "<gyro>"
  [Sen] -> Bus Selector2/1
  Selector2/1 -> [b_est]

== system Two_Attitude_Estimation_ekf/Quad with sensors+estimator/Attitude representation ==
  note: nomenclature
      | gRb implies: gv = gRb * bv
      | bRg implies: bv = bRg * gv
      |
      | wb = angular velocity expressed in components of the B-frame
      | gwb = angular velocity expressed in components of the G-frame
  q_est : Inport
  Calc Euler_rates : Subsystem
  MATLAB Function2 : MATLAB Function  TreatAsAtomicUnit=on
  Mux : Mux  Inputs=3
  Quaternion Normalize : sharedutil/Quaternion Normalize  aMode=aMode
      settings: SourceProductBaseCode=AE,PW,DR,MT,UV,VE
  Quaternions to Direction Cosine Matrix : sharedtransform/Quaternions to  Direction Cosine Matrix  Commented=on  aMode=aMode
      settings: SourceProductBaseCode=AE,PW,DR,MT,UV,VE
  Reshape1 : Reshape  OutputDimensionality=Column vector (2-D)
  calc_bRg : MATLAB Function  TreatAsAtomicUnit=on
  Euler_rates : Outport
  bRg : Outport  Port=2
  Euler : Outport  Port=3
  wires:
  Calc Euler_rates/1(Euler_rates) -> Euler_rates/1
  [Eul] -> Calc Euler_rates/2(Euler_angs)
  [wb] -> Calc Euler_rates/1("p q r ")
  Reshape1/1 -> [Eul], Euler/1
  Mux/1 -> Reshape1/1
  MATLAB Function2/3(psi) -> Mux/3
  MATLAB Function2/2(theta) -> Mux/2
  MATLAB Function2/1(phi) -> Mux/1
  calc_bRg/1(bRg) -> bRg/1, MATLAB Function2/1(R), [bRg]  "bRg"
  q_est/1 -> Quaternion Normalize/1
  Quaternion Normalize/1 -> [q], calc_bRg/1(q)

== system Two_Attitude_Estimation_ekf/Quad_EOM/Gravity_G_to_B ==
  note: F_B = ^BR_G * F_G
  bRg : Inport
  Product : Product  Multiplication=Matrix(*)
  Product1 : Product
  gravity vector in inertial frame : Constant  Value=[0;0;g]  VectorParams1D=off
  mass : Constant  Value=m
  Fb_gravity : Outport  VectorParamsAs1DForOutWhenUnconnected=off
  wires:
  bRg/1 -> Product/1
  Product/1 -> Fb_gravity/1  "F_garvity in body frame"
  Product1/1 -> Product/2  "m*g"
  gravity vector in inertial frame/1 -> Product1/1  "Fg"
  mass/1 -> Product1/2

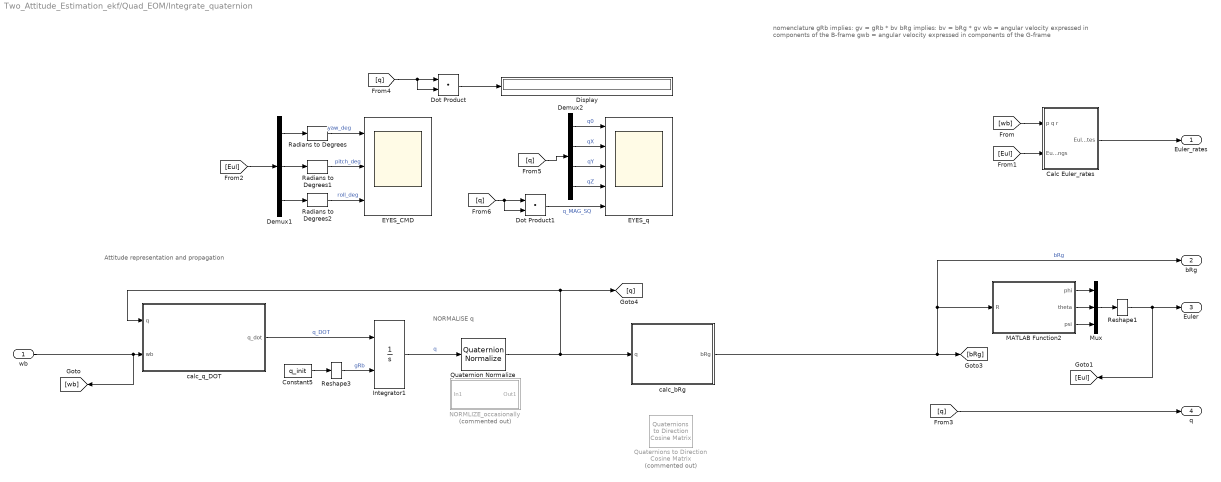
== system Two_Attitude_Estimation_ekf/Quad_EOM/Integrate_quaternion ==
  note: Attitude representation and propagation
  note: nomenclature
      | gRb implies: gv = gRb * bv
      | bRg implies: bv = bRg * gv
      |
      | wb = angular velocity expressed in components of the B-frame
      | gwb = angular velocity expressed in components of the G-frame
  note: NORMALISE q
  wb : Inport
  Calc Euler_rates : Subsystem
  Constant5 : Constant  Value=q_init  OutDataTypeStr=Inherit: Inherit via back propagation
  Demux1 : Demux  Outputs=3
  Demux2 : Demux
  Display : Display
  Dot Product : DotProduct  InputSameDT=on  OutDataTypeStr=Inherit: Inherit via internal rule
  Dot Product1 : DotProduct  InputSameDT=on  OutDataTypeStr=Inherit: Inherit via internal rule
  EYES_CMD : Scope  NumInputPorts=3
  EYES_q : Scope  NumInputPorts=5
  Integrator1 : Integrator  InitialConditionSource=external
  MATLAB Function2 : MATLAB Function  TreatAsAtomicUnit=on
  Mux : Mux  Inputs=3
  NORMLIZE_occasionally : Subsystem  Commented=on
  Quaternion Normalize : sharedutil/Quaternion Normalize  aMode=aMode
      settings: SourceProductBaseCode=AE,PW,DR,MT,UV,VE
  Quaternions to Direction Cosine Matrix : sharedtransform/Quaternions to  Direction Cosine Matrix  Commented=on  aMode=aMode
      settings: SourceProductBaseCode=AE,PW,DR,MT,UV,VE
  Radians to Degrees : simulink_extras/Transformations/Radians to Degrees
  Radians to Degrees1 : simulink_extras/Transformations/Radians to Degrees
  Radians to Degrees2 : simulink_extras/Transformations/Radians to Degrees
  Reshape1 : Reshape  OutputDimensionality=Column vector (2-D)
  Reshape3 : Reshape  OutputDimensionality=Column vector (2-D)
  calc_bRg : MATLAB Function  TreatAsAtomicUnit=on
  calc_q_DOT : MATLAB Function  TreatAsAtomicUnit=on
  Euler_rates : Outport
  bRg : Outport  Port=2
  Euler : Outport  Port=3
  q : Outport  Port=4
  wires:
  Calc Euler_rates/1(Euler_rates) -> Euler_rates/1
  [Eul] -> Demux1/1
  Demux1/2 -> Radians to Degrees1/1
  Demux1/3 -> Radians to Degrees2/1
  Radians to Degrees2/1 -> EYES_CMD/3  "roll_deg"
  Radians to Degrees1/1 -> EYES_CMD/2  "pitch_deg"
  Radians to Degrees/1 -> EYES_CMD/1  "yaw_deg"
  Demux1/1 -> Radians to Degrees/1
  [Eul] -> Calc Euler_rates/2(Euler_angs)
  [wb] -> Calc Euler_rates/1("p q r ")
  Reshape1/1 -> [Eul], Euler/1
  Mux/1 -> Reshape1/1
  MATLAB Function2/3(psi) -> Mux/3
  MATLAB Function2/2(theta) -> Mux/2
  MATLAB Function2/1(phi) -> Mux/1
  Demux2/3 -> EYES_q/3  "qY"
  [q] -> Demux2/1
  Demux2/2 -> EYES_q/2  "qX"
  Demux2/1 -> EYES_q/1  "q0"
  [q] -> Dot Product1/2, Dot Product1/1
  Demux2/4 -> EYES_q/4  "qZ"
  Dot Product1/1 -> EYES_q/5  "q_MAG_SQ"
  Dot Product/1 -> Display/1
  [q] -> Dot Product/2, Dot Product/1
  Integrator1/1 -> Quaternion Normalize/1  "q"
  Quaternion Normalize/1 -> calc_bRg/1(q), [q], calc_q_DOT/1(q)
  calc_bRg/1(bRg) -> bRg/1, MATLAB Function2/1(R), [bRg]  "bRg"
  calc_q_DOT/1(q_dot) -> Integrator1/1  "q_DOT"
  Constant5/1 -> Reshape3/1
  wb/1 -> calc_q_DOT/2(wb), [wb]
  Reshape3/1 -> Integrator1/2  "gRb"
  [q] -> q/1

== system Two_Attitude_Estimation_ekf/Quad_EOM/Subsystem ==
  note: I . w^' = Mb - (\omega \times (I.w))
      |
      | w^' = inv(I) * (Mb - (w \times (I.w)))
  pqr : Inport
  I : Inport  Port=2
  Moment : Inport  Port=3
  Product2 : Product  Multiplication=Matrix(*)  InputSameDT=on  SaturateOnIntegerOverflow=on  OutDataTypeStr=Inherit: Same as first input
  Product3 : Product  Inputs=/  Multiplication=Matrix(*)  SaturateOnIntegerOverflow=on  OutDataTypeStr=Inherit: Same as first input
  Product4 : Product  Multiplication=Matrix(*)  SaturateOnIntegerOverflow=on  OutDataTypeStr=Inherit: Same as first input
  Reshape10 : Reshape  OutputDimensionality=Column vector (2-D)
  Reshape8 : Reshape  OutputDimensionality=Column vector (2-D)
  Reshape9 : Reshape  OutputDimensionality=Column vector (2-D)
  Scope : Scope
  Scope1 : Scope
  Scope2 : Scope
  Sum2 : Sum  Inputs=+|-  SaturateOnIntegerOverflow=on
  w_x_(I.w) : Subsystem
      mask Display:
      | text(.5,.5,'Cross\nProduct\n\nC = AxB', ...
      | 	'HorizontalAlignment','Center',...
      | 	'VerticalAlignment','middle')
  pdot qdot rdot : Outport
  wires:
  Product2/1 -> Scope1/1, w_x_(I.w)/2(B)  "I.w"
  Product3/1 -> Product4/1  "inv(I)"
  Reshape8/1 -> Scope/1, w_x_(I.w)/1(A), Product2/2  "w"
  [I] -> Product3/1
  pqr/1 -> Reshape8/1
  Reshape9/1 -> Sum2/1  "Mb"
  Sum2/1 -> Scope2/1, Product4/2  "Mb - (w x (I.w))"
  Reshape10/1 -> Sum2/2  "w x (I.w)"
  w_x_(I.w)/1(C) -> Reshape10/1
  [I] -> Product2/1  "I"
  Product4/1 -> pdot qdot rdot/1  "w_dot"
  Moment/1 -> Reshape9/1
  I/1 -> [I]

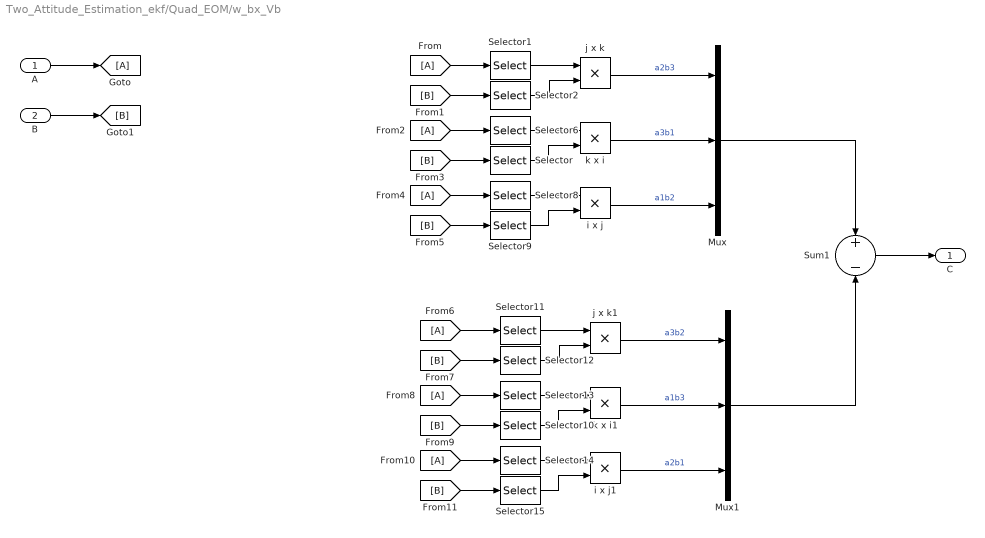
== system Two_Attitude_Estimation_ekf/Quad_EOM/w_bx_Vb ==
  A : Inport
  B : Inport  Port=2
  Mux : Mux  Inputs=3
  Mux1 : Mux  Inputs=3
  Selector{,8,13,15} (4 alike) : Selector  InputPortWidth=3  IndexOptions=Index vector (dialog)  Indices=1  OutputSizes=1
  Selector{1,9,12,14} (4 alike) : Selector  InputPortWidth=3  IndexOptions=Index vector (dialog)  Indices=2  OutputSizes=1
  Selector{2,6,10..11} (4 alike) : Selector  InputPortWidth=3  IndexOptions=Index vector (dialog)  Indices=3  OutputSizes=1
  Sum1 : Sum  Inputs=+|-  InputSameDT=on  SaturateOnIntegerOverflow=on  OutDataTypeStr=Inherit: Same as first input
  i x j : Product  InputSameDT=on  SaturateOnIntegerOverflow=on  OutDataTypeStr=Inherit: Same as first input
  i x j1 : Product  InputSameDT=on  SaturateOnIntegerOverflow=on  OutDataTypeStr=Inherit: Same as first input
  j x k : Product  InputSameDT=on  SaturateOnIntegerOverflow=on  OutDataTypeStr=Inherit: Same as first input
  j x k1 : Product  InputSameDT=on  SaturateOnIntegerOverflow=on  OutDataTypeStr=Inherit: Same as first input
  k x i : Product  InputSameDT=on  SaturateOnIntegerOverflow=on  OutDataTypeStr=Inherit: Same as first input
  k x i1 : Product  InputSameDT=on  SaturateOnIntegerOverflow=on  OutDataTypeStr=Inherit: Same as first input
  C : Outport
  wires:
  i x j/1 -> Mux/3  "a1b2"
  k x i/1 -> Mux/2  "a3b1"
  j x k/1 -> Mux/1  "a2b3"
  Mux/1 -> Sum1/1
  Sum1/1 -> C/1
  Selector1/1 -> j x k/1
  Selector2/1 -> j x k/2
  B/1 -> [B]
  A/1 -> [A]
  [B] -> Selector2/1
  [A] -> Selector1/1
  [A] -> Selector6/1
  [B] -> Selector/1
  Selector6/1 -> k x i/1
  Selector/1 -> k x i/2
  [A] -> Selector8/1
  [B] -> Selector9/1
  Selector8/1 -> i x j/1
  Selector9/1 -> i x j/2
  i x j1/1 -> Mux1/3  "a2b1"
  k x i1/1 -> Mux1/2  "a1b3"
  j x k1/1 -> Mux1/1  "a3b2"
  Mux1/1 -> Sum1/2
  Selector11/1 -> j x k1/1
  Selector12/1 -> j x k1/2
  [B] -> Selector12/1
  [A] -> Selector11/1
  [A] -> Selector13/1
  [B] -> Selector10/1
  Selector13/1 -> k x i1/1
  Selector10/1 -> k x i1/2
  [A] -> Selector14/1
  [B] -> Selector15/1
  Selector14/1 -> i x j1/1
  Selector15/1 -> i x j1/2

== system Two_Attitude_Estimation_ekf/Sensors and preprocessing/IMU+altitude ==
  note: Accelerometer and Gyroscope
  note: Magnetometer
  note: Altitude (not simulated)
  States : Inport
  Acc + Gyro : Subsystem  AncestorBlock=aerolibnav/Three-axis Inertial Measurement Unit  mask(Three-axis Inertial Measurement Unit){units=Metric (MKS), imu=[0 0 0], i_Ts=Ts, dtype_a=off, w_a=.7, z_a=.2, a_sf_cc=IMU.accScaleCross, a_bias=IMU.accBias, a_sat=IMU.accLimits, dtype_g=off, w_g=.7, z_g=.2, g_sf_cc=IMU.gyroScaleCross, g_bias=IMU.gyroBias, g_sens=[0, 0, 0], g_sat=IMU.gyroLimits, i_rand=on, i_seeds=IMU.noiseSeeds, i_pow=IMU.noisePower}
      mask prompts: units "aeroblks:aeroblknav:blockThreeaxisInertialMeasurementUnitParamUnits"; imu "aeroblks:aeroblknav:blockThreeaxisInertialMeasurementUnitParamIMUlocation"; i_Ts "aeroblks:aeroblknav:blockThreeaxisInertialMeasurementUnitParamUpdaterate"; dtype_a "aeroblks:aeroblknav:blockThreeaxisInertialMeasurementUnitParamSecondorderdynamicsforaccelerometer"; w_a "aeroblks:aeroblknav:blockThreeaxisInertialMeasurementUnitParamAccelerometernaturalfrequencyradsec"; z_a "aeroblks:aeroblknav:blockThreeaxisInertialMeasurementUnitParamAccelerometerdampingratio"; a_sf_cc "aeroblks:aeroblknav:blockThreeaxisInertialMeasurementUnitParamAccelerometerscalefactorandcrosscoupling"; a_bias "aeroblks:aeroblknav:blockThreeaxisInertialMeasurementUnitParamAccelerometermeasurementbias"; a_sat "aeroblks:aeroblknav:blockThreeaxisInertialMeasurementUnitParamAccelerometerupperandlowerlimits"; dtype_g "aeroblks:aeroblknav:blockThreeaxisInertialMeasurementUnitParamSecondorderdynamicsforgyro"; w_g "aeroblks:aeroblknav:blockThreeaxisInertialMeasurementUnitParamGyronaturalfrequencyradsec"; z_g "aeroblks:aeroblknav:blockThreeaxisInertialMeasurementUnitParamGyrodampingratio"; g_sf_cc "aeroblks:aeroblknav:blockThreeaxisInertialMeasurementUnitParamGyroscalefactorsandcrosscoupling"; g_bias "aeroblks:aeroblknav:blockThreeaxisInertialMeasurementUnitParamGyromeasurementbias"; g_sens "aeroblks:aeroblknav:blockThreeaxisInertialMeasurementUnitParamGsensitivebias"; g_sat "aeroblks:aeroblknav:blockThreeaxisInertialMeasurementUnitParamGyroupperandlowerlimits"; i_rand "aeroblks:aeroblknav:blockThreeaxisInertialMeasurementUnitParamNoiseon"; i_seeds "aeroblks:aeroblknav:blockThreeaxisInertialMeasurementUnitParamNoiseseeds"; i_pow "aeroblks:aeroblknav:blockThreeaxisInertialMeasurementUnitParamNoisepower"
      mask help: aeroblks:aeroblknav:blockThreeaxisInertialMeasurementUnitDesc
      mask init:
      | block = gcb;   
      | ports=aeroicon('aeroblkimu','icon');
      mask Help: eval('asbhelp');
      mask TypeOptions units: aeroblks:aeroblknav:blockThreeaxisInertialMeasurementUnitParamComboMetricMKS | aeroblks:aeroblknav:blockThreeaxisInertialMeasurementUnitParamComboEnglish
      mask Callback dtype_a: aeroicon('aeroblkimu')
      mask Callback dtype_g: aeroicon('aeroblkimu')
      mask Callback i_rand: aeroicon('aeroblkimu')
      mask DialogControl ParameterTabVar0 Prompt: Main
      mask DialogControl units Prompt: Units:
      mask DialogControl imu Prompt: IMU location:
      mask DialogControl i_Ts Prompt: Update rate:
      mask DialogControl ParameterTabVar01 Prompt: Accelerometer
      mask DialogControl dtype_a Prompt: Second-order dynamics for accelerometer
      mask DialogControl w_a Prompt: Accelerometer natural frequency (rad/sec):
      mask DialogControl z_a Prompt: Accelerometer damping ratio:
      mask DialogControl a_sf_cc Prompt: Accelerometer scale factor and cross-coupling:
      mask DialogControl a_bias Prompt: Accelerometer measurement bias:
      mask DialogControl a_sat Prompt: Accelerometer upper and lower limits:
      mask DialogControl ParameterTabVar012 Prompt: Gyroscope
      mask DialogControl dtype_g Prompt: Second-order dynamics for gyro
      mask DialogControl w_g Prompt: Gyro natural frequency (rad/sec):
      mask DialogControl z_g Prompt: Gyro damping ratio:
      mask DialogControl g_sf_cc Prompt: Gyro scale factors and cross-coupling:
      mask DialogControl g_bias Prompt: Gyro measurement bias:
      mask DialogControl g_sens Prompt: G-sensitive bias:
      mask DialogControl g_sat Prompt: Gyro upper and lower limits:
      mask DialogControl ParameterTabVar0123 Prompt: Noise
      mask DialogControl i_rand Prompt: Noise on
      mask DialogControl i_seeds Prompt: Noise seeds:
      mask DialogControl i_pow Prompt: Noise power:
      mask Display:
      | port_label(ports(1).type,ports(1).port,ports(1).txt,'texmode','on');
      | port_label(ports(2).type,ports(2).port,ports(2).txt,'texmode','on');
      | port_label(ports(3).type,ports(3).port,ports(3).txt,'texmode','on');
      | port_label(ports(4).type,ports(4).port,ports(4).txt,'texmode','on');
      | port_label(ports(5).type,ports(5).port,ports(5).txt,'texmode','on');
      | port_label(ports(6).type,ports(6).port,ports(6).txt,'texmode','on');
      | port_label(ports(7).type,ports(7).port,ports(7).txt,'texmode','on');
  Bus Selector : BusSelector  OutputSignals=Ab,wb,wb_dot
  Bus Selector1 : BusSelector  OutputSignals=Ab,bRg
  Bus Selector3 : BusSelector  OutputSignals=phi; theta; psi
  Bus Selector4 : BusSelector  OutputSignals=Xe
  Bus Selector5 : BusSelector  OutputSignals=Ab
  CG location : Constant  Value=[0, 0, 0]
  Compare yaw from mag and actual one : MATLAB Function  TreatAsAtomicUnit=on
  Gravity : Constant  Value=[0 0 -g]
  IMU : mspsensorlib/IMU  Commented=on  DispRefFrame=NED  Temperature=25  MagneticFieldNED=[ 27.5550, -2.4169, -16.0849 ]  MagneticFieldENU=[ -2.4169, 27.5550, 16.0849 ]  SeedDouble=67  SimulateUsing=Interpreted execution  AccelParamsMeasurementRange=Inf  AccelParamsResolution=0  AccelParamsConstantBias=[ 0, 0, 0 ]  AccelParamsAxesMisalignment=[ 0, 0, 0 ]  AccelParamsNoiseDensity=[ 0, 0, 0 ]  AccelParamsBiasInstability=[ 0, 0, 0 ]  AccelParamsRandomWalk=[ 0, 0, 0 ]  AccelParamsTemperatureBias=[ 0, 0, 0 ]  AccelParamsTemperatureScaleFactor=[ 0, 0, 0 ]  GyroParamsMeasurementRange=Inf  GyroParamsResolution=0  GyroParamsConstantBias=[ 0, 0, 0 ]  GyroParamsAxesMisalignment=[ 0, 0, 0 ]  GyroParamsAccelerationBias=[ 0, 0, 0 ]  GyroParamsNoiseDensity=[ 0, 0, 0 ]  GyroParamsBiasInstability=[ 0, 0, 0 ]  GyroParamsRandomWalk=[ 0, 0, 0 ]  GyroParamsTemperatureBias=[ 0, 0, 0 ]  GyroParamsTemperatureScaleFactor=[ 0, 0, 0 ]  MagParamsMeasurementRange=Inf  MagParamsResolution=0  MagParamsConstantBias=[ 0, 0, 0 ]  MagParamsAxesMisalignment=[ 0, 0, 0 ]  MagParamsNoiseDensity=[ 0, 0, 0 ]  MagParamsBiasInstability=[ 0, 0, 0 ]  MagParamsRandomWalk=[ 0, 0, 0 ]  MagParamsTemperatureBias=[ 0, 0, 0 ]  MagParamsTemperatureScaleFactor=[ 0, 0, 0 ]
      settings: SourceProductBaseCode=TF,NV
  Magnetometer : Subsystem
  Mux : Mux  Inputs=2
  Scope : Scope
  Selector : Selector  InputPortWidth=3  IndexOptions=Index vector (dialog)  Indices=[3]  OutputSizes=1
  Selector2 : Selector  InputPortWidth=3  IndexOptions=Index vector (dialog)  Indices=[3]  OutputSizes=1
  Three-axis Inertial Measurement Unit1 : aerolibnav/Three-axis Inertial Measurement Unit  Commented=on  units=Metric (MKS)  imu=[0 0 0]  i_Ts=Ts_IMU  dtype_a=on  w_a=190  z_a=0.707  a_sf_cc=[1 0 0; 0 1 0; 0 0 1]  a_bias=[0 0 0]  a_sat="[-inf  -inf  -inf  inf inf inf]"  dtype_g=on  w_g=190  z_g=0.707  g_sf_cc=[1 0 0; 0 1 0; 0 0 1]  g_bias=[0 0 0]  g_sens=[0 0 0]  g_sat="[-inf  -inf  -inf  inf inf inf]"  i_rand=on  i_seeds=[23093 23094 23095 23096 23097 23098]  i_pow=[0.001 0.001 0.001 0.0001 0.0001 0.0001]
  acc : Outport
  gyro : Outport  Port=2
  alt : Outport  Port=3
  mag : Outport  Port=4
  wires:
  Selector2/1 -> alt/1  "altitude"
  CG location/1 -> Acc + Gyro/4(CG)
  Bus Selector/3 -> Acc + Gyro/3(w_dot)  "<wb_dot>"
  Bus Selector/2 -> Acc + Gyro/2(w)  "<wb>"
  Bus Selector/1 -> Acc + Gyro/1(A_b)  "<Ab>"
  Acc + Gyro/2(w_meas) -> gyro/1  "gyro"
  Gravity/1 -> Acc + Gyro/5(g)  "Gravity_ned"
  Acc + Gyro/1(A_meas) -> acc/1  "acc"
  Selector/1 -> Mux/2  "yaw"
  Compare yaw from mag and actual one/1(yaw) -> Mux/1
  Mux/1 -> Scope/1
  Bus Selector1/2 -> Magnetometer/2(<bRg>)  "<bRg>"
  Magnetometer/1(mag) -> mag/1, Compare yaw from mag and actual one/2(mag_vec)
  States/1 -> [states]
  [states] -> Bus Selector/1
  [states] -> Bus Selector1/1
  [states] -> Bus Selector3/1
  Bus Selector3/1 -> Selector/1  "<phi; theta; psi>"
  [states] -> Bus Selector4/1
  Bus Selector4/1 -> Selector2/1  "<Xe>"
  Bus Selector1/1 -> Magnetometer/1(acc)  "<Ab>"
  [states] -> Bus Selector5/1
  Bus Selector5/1 -> Compare yaw from mag and actual one/1(acc_vec)  "<Ab>"

== system Two_Attitude_Estimation_ekf/Sensors and preprocessing/Preprocessing and Filtering ==
  acc_raw : Inport
  gyro_raw : Inport  Port=2
  alt_raw : Inport  Port=3
  mag_raw : Inport  Port=4
  Cast To Double{,1..2,4} (4 alike) : DataTypeConversion  OutDataTypeStr=double
  Constant : Constant  Value=[0 0 g]
  FIR_IMUaccel : DiscreteFir  Coefficients=accel_filter_coef
  IIR_IMUgyro : DiscreteFilter  Numerator=gyro_filter_num  Denominator=gyro_filter_den
  Sum : Sum  Inputs=-+|
  Sum1 : Sum  Inputs=-+|
  Sum2 : Sum  Inputs=-+|
  Sum3 : Sum  Inputs=|+-
  bias : Constant  Value=IMU.accBiasEst
  filtering : Subsystem
  gyro bias : Constant  Value=IMU.gyroBiasEst
  inverseI_acc_gain : Gain  Gain=IMU.inverseAccGain  ParamDataTypeStr=single  OutDataTypeStr=single
  inverseI_gyro_gain : Gain  Gain=IMU.inverseGyroGain  ParamDataTypeStr=single  OutDataTypeStr=single
  inverseI_mag_gain : Gain  Gain=IMU.inverseMagGain  ParamDataTypeStr=single  OutDataTypeStr=single
  mag bias : Constant  Value=IMU.magBiasEst
  acc_zero : Outport
  acc : Outport  Port=2
  gyro : Outport  Port=3
  alt : Outport  Port=4
  mag : Outport  Port=5
  wires:
  gyro bias/1 -> Sum2/1
  Cast To Double/1 -> acc/1, Sum/2  "acc"
  bias/1 -> Sum1/1
  mag bias/1 -> Sum3/2
  FIR_IMUaccel/1 -> Cast To Double/1  "acc"
  inverseI_gyro_gain/1 -> filtering/1(gyro_raw)  "gyro"
  mag_raw/1 -> Sum3/1
  Sum3/1 -> inverseI_mag_gain/1  "gyro"
  Sum1/1 -> inverseI_acc_gain/1  "acc"
  Sum/1 -> acc_zero/1  "acc_zero"
  Sum2/1 -> inverseI_gyro_gain/1  "gyro"
  Cast To Double1/1 -> gyro/1  "gyro"
  inverseI_mag_gain/1 -> IIR_IMUgyro/1  "mag"
  IIR_IMUgyro/1 -> Cast To Double4/1
  filtering/1(gyro) -> Cast To Double1/1  "gyro"
  inverseI_acc_gain/1 -> FIR_IMUaccel/1  "acc"
  Cast To Double4/1 -> mag/1  "mag"
  Constant/1 -> Sum/1
  acc_raw/1 -> Sum1/2
  gyro_raw/1 -> Sum2/2
  Cast To Double2/1 -> alt/1  "alt"
  alt_raw/1 -> Cast To Double2/1
